simulink model "Powertrain"  (R2025b)
settings: Solver=FixedStepAuto  StartTime=0.0  StopTime=10.0  FixedStep=1e-3  RelTol=1e-3
settings Model: Creator=nikol  LastModifiedBy=nikol

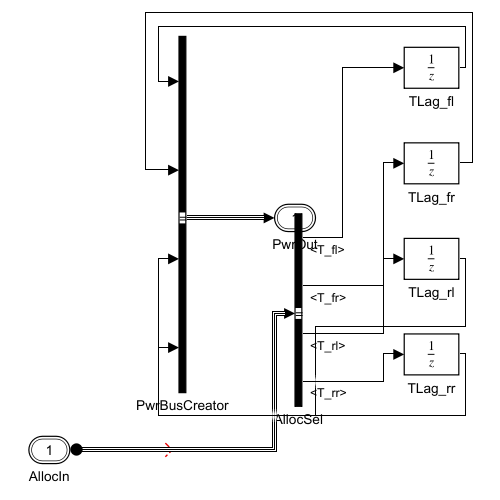
[thumbnail: Simulink's stored preview of the top-level diagram]
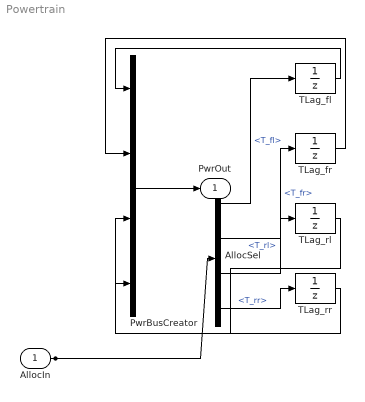
== system Powertrain ==
  AllocIn : Inport  OutDataTypeStr=Bus: AllocBus
  AllocSel : BusSelector  OutputSignals=T_fl,T_fr,T_rl,T_rr
  PwrBusCreator : BusCreator  Inputs=4  OutDataTypeStr=Bus: PwrBus
      settings: InheritFromInputs=off
  TLag_fl : UnitDelay  SampleTime=-1  HasFrameUpgradeWarning=on
  TLag_fr : UnitDelay  SampleTime=-1  HasFrameUpgradeWarning=on
  TLag_rl : UnitDelay  SampleTime=-1  HasFrameUpgradeWarning=on
  TLag_rr : UnitDelay  SampleTime=-1  HasFrameUpgradeWarning=on
  PwrOut : Outport  OutDataTypeStr=Bus: PwrBus
  wires:
  AllocIn/1 -> AllocSel/1
  PwrBusCreator/1 -> PwrOut/1
  AllocSel/1 -> TLag_fl/1  "<T_fl>"
  TLag_fl/1 -> PwrBusCreator/1
  AllocSel/2 -> TLag_fr/1  "<T_fr>"
  TLag_fr/1 -> PwrBusCreator/2
  AllocSel/3 -> TLag_rl/1  "<T_rl>"
  TLag_rl/1 -> PwrBusCreator/3
  AllocSel/4 -> TLag_rr/1  "<T_rr>"
  TLag_rr/1 -> PwrBusCreator/4
